simulink model "ACC_Model1"  (R2026a)
settings: Solver=ode45  StopTime=60  RelTol=1e-4
libraries: slpidlib x1
settings Model: Creator=walis  LastModifiedBy=walis
settings DebuggingCC: InheritedTsInSrcMsg=none

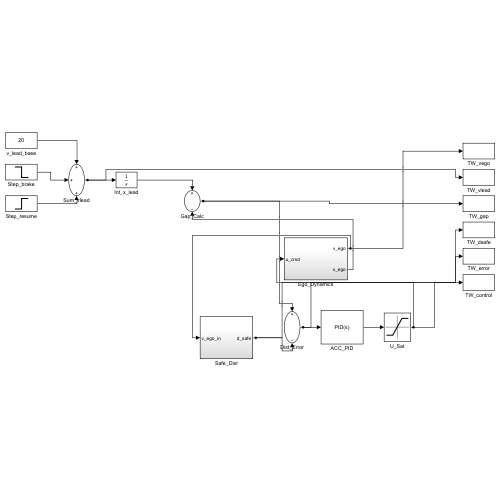
[thumbnail: Simulink's stored preview of the top-level diagram]
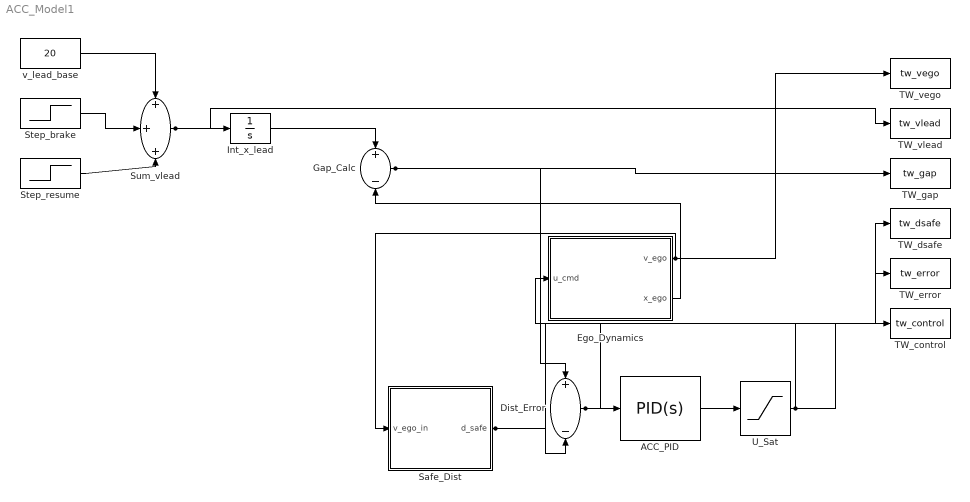
== system ACC_Model1 ==
  ACC_PID : slpidlib/PID Controller  Controller=PID  Form=Parallel  TimeDomain=Continuous-time  UseExternalTs=off  SampleTime=-1  IntegratorMethod=Forward Euler  FilterMethod=Forward Euler  ControllerParametersSource=internal  P=200  I=5  UseKiTs=off  D=50  UseExternalDerivativeSource=off  N=100  UseFilter=on  TunerSelectOption=Transfer Function Based (PID Tuner App)  InitialConditionSource=internal  InitialConditionForIntegrator=0  InitialConditionForFilter=0  DifferentiatorICPrevScaledInput=0  ExternalReset=none  TrackingMode=off  Kt=1  LimitOutput=off  SatLimitsSource=internal  UpperSaturationLimit=inf  LowerSaturationLimit=-inf  LinearizeAsGain=on  AntiWindupMode=none  Kb=1  LimitIntegrator=off  UpperIntegratorSaturationLimit=inf  LowerIntegratorSaturationLimit=-inf  POutMin=[]  POutMax=[]  IOutMin=[]  IOutMax=[]  DOutMin=[]  DOutMax=[]  NOutMin=[]  NOutMax=[]  SumOutMin=[]  SumOutMax=[]  SaturationOutMin=[]  SaturationOutMax=[]  PParamMin=[]  PParamMax=[]  IParamMin=[]  IParamMax=[]  DParamMin=[]  DParamMax=[]  NParamMin=[]  NParamMax=[]  KbParamMin=[]  KbParamMax=[]  KtParamMin=[]  KtParamMax=[]  KbOutMin=[]  KbOutMax=[]  KtOutMin=[]  KtOutMax=[]  IntegratorOutMin=[]  IntegratorOutMax=[]  FilterOutMin=[]  FilterOutMax=[]  SumI1OutMin=[]  SumI1OutMax=[]  SumI2OutMin=[]  SumI2OutMax=[]  SumI3OutMin=[]  SumI3OutMax=[]  SumI4OutMin=[]  SumI4OutMax=[]  SumDOutMin=[]  SumDOutMax=[]  DifferentiatorOutMin=[]  DifferentiatorOutMax=[]  FilterDiffOutCoefMin=[]  FilterDiffOutCoefMax=[]  ReciprocalOutMin=[]  ReciprocalOutMax=[]  SumDenOutMin=[]  SumDenOutMax=[]  SumNumOutMin=[]  SumNumOutMax=[]  DivideOutMin=[]  DivideOutMax=[]  UdiffTsProdOutMin=[]  UdiffTsProdOutMax=[]  NTsProdOutMin=[]  NTsProdOutMax=[]  UintegralTsProdOutMin=[]  UintegralTsProdOutMax=[]  UngainTsProdOutMin=[]  UngainTsProdOutMax=[]  ClampingZeroOutDataTypeStr=Inherit: Inherit via back propagation  ClampingZeroOutMin=[]  ClampingZeroOutMax=[]  FilterDenConstantOutDataTypeStr=Inherit: Inherit via back propagation  FilterDenConstantOutMin=[]  FilterDenConstantOutMax=[]  PCopyOutDataTypeStr=Inherit: Inherit via back propagation  PCopyOutMin=[]  PCopyOutMax=[]  NCopyOutDataTypeStr=Inherit: Inherit via back propagation  NCopyOutMin=[]  NCopyOutMax=[]  IntegratorContinuousStateAttributes=''  IntegratorStateMustResolveToSignalObject=off  IntegratorRTWStateStorageClass=Auto  FilterContinuousStateAttributes=''  FilterStateMustResolveToSignalObject=off  FilterRTWStateStorageClass=Auto  ParallelPVariant=InternalParameters  IdealPVariant=Disabled  IVariant=InternalParameters  DVariant=InternalParameters  IntegratorVariant=Continuous  SatVariant=Disabled  AWVariant=Passthrough  PCopyVariant=Disabled  TRVariant=Disabled  FdbkBlocksVariant=Forward  IdealPFdbkVariant=Disabled  SatFdbkVariant=Disabled  DerivativeFilterVariant=ContFilter  NVariant=InternalParameters  NCopyVariant=Disabled  FilterICVariant=InternalICsFilter  IntegratorICVariant=InternalICs  ExternalResetVariant=Disabled  TRSumVariant=Passthrough  SumFdbkVariant=Disabled  SumVariant=Sum_PID  TsampFilterVariant=InternalTs  TsampNgainVariant=Passthrough  TsampIntegralVariant=Disabled_SignalSpec  ExternalSaturationOutDataTypeStr=Inherit: Same as second input  DerivativeSourceVariant=ErrorSignal  PreIntVariant=InternalPreInt
  Dist_Error : Sum  Inputs=+-
  Ego_Dynamics : Subsystem
  Gap_Calc : Sum  Inputs=+-
  Int_x_lead : Integrator  InitialCondition=40
  Safe_Dist : Subsystem
  Step_brake : Step  Time=10  FinalValue=-10  SampleTime=0
  Step_resume : Step  Time=35  FinalValue=10  SampleTime=0
  Sum_vlead : Sum  Inputs=+++
  TW_control : ToWorkspace  VariableName=tw_control  SampleTime=-1
  TW_dsafe : ToWorkspace  VariableName=tw_dsafe  SampleTime=-1
  TW_error : ToWorkspace  VariableName=tw_error  SampleTime=-1
  TW_gap : ToWorkspace  VariableName=tw_gap  SampleTime=-1
  TW_vego : ToWorkspace  VariableName=tw_vego  SampleTime=-1
  TW_vlead : ToWorkspace  VariableName=tw_vlead  SampleTime=-1
  U_Sat : Saturate  UpperLimit=3000  LowerLimit=-3000
  v_lead_base : Constant  Value=20  SampleTime=0
  wires:
  v_lead_base/1 -> Sum_vlead/1
  Step_brake/1 -> Sum_vlead/2
  Step_resume/1 -> Sum_vlead/3
  Sum_vlead/1 -> Int_x_lead/1, TW_vlead/1
  Int_x_lead/1 -> Gap_Calc/1
  Ego_Dynamics/2(x_ego) -> Gap_Calc/2
  Ego_Dynamics/1(v_ego) -> Safe_Dist/1(v_ego_in), TW_vego/1
  Gap_Calc/1 -> Dist_Error/1, TW_gap/1
  Safe_Dist/1(d_safe) -> Dist_Error/2, TW_dsafe/1
  Dist_Error/1 -> ACC_PID/1, TW_error/1
  ACC_PID/1 -> U_Sat/1
  U_Sat/1 -> Ego_Dynamics/1(u_cmd), TW_control/1

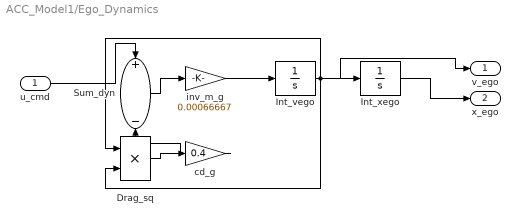
== system ACC_Model1/Ego_Dynamics ==
  u_cmd : Inport
  Drag_sq : Product
  Int_vego : Integrator  InitialCondition=20
  Int_xego : Integrator
  Sum_dyn : Sum  Inputs=+-
  cd_g : Gain  Gain=0.4
  inv_m_g : Gain  Gain=0.00066667
  v_ego : Outport
  x_ego : Outport  Port=2
  wires:
  u_cmd/1 -> Sum_dyn/1
  Sum_dyn/1 -> inv_m_g/1
  inv_m_g/1 -> Int_vego/1
  Int_vego/1 -> Int_xego/1, Drag_sq/1, Drag_sq/2, v_ego/1
  Drag_sq/1 -> cd_g/1
  cd_g/1 -> Sum_dyn/2
  Int_xego/1 -> x_ego/1

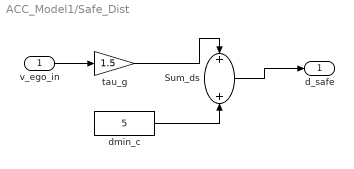
== system ACC_Model1/Safe_Dist ==
  v_ego_in : Inport
  Sum_ds : Sum
  dmin_c : Constant  Value=5  SampleTime=0
  tau_g : Gain  Gain=1.5
  d_safe : Outport
  wires:
  v_ego_in/1 -> tau_g/1
  tau_g/1 -> Sum_ds/1
  dmin_c/1 -> Sum_ds/2
  Sum_ds/1 -> d_safe/1
